simulink model "ASK_SIM"  (R2024a)
settings: Solver=VariableStepAuto  StartTime=0.0  StopTime=10.0  RelTol=1e-3
libraries: commrandsrc3 x1
settings Model: Creator=adity  LastModifiedBy=adity

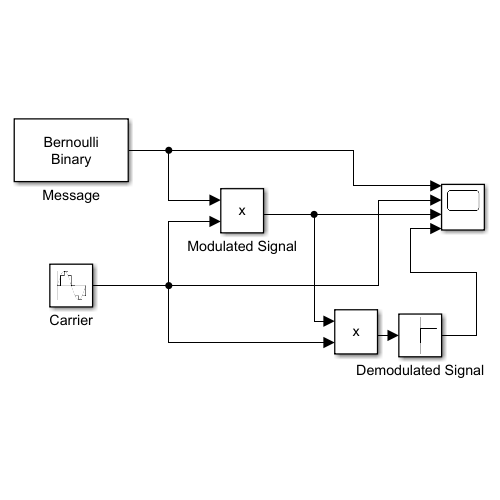
[thumbnail: Simulink's stored preview of the top-level diagram]
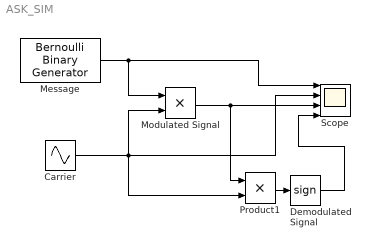
== system ASK_SIM ==
  Carrier : Sin  Frequency=2*pi*5  SampleTime=1/1000  VectorParams1D=off
  Demodulated Signal : Signum
  Message : commrandsrc3/Bernoulli Binary Generator  ProbabilityOfZero=0.5  SeedSource=Auto  Seed=0  SampleTime=0.5  SamplesPerFrame=1  OutputDataType=double  SimulateUsing=Interpreted execution
  Modulated Signal : Product
  Product1 : Product
  Scope : Scope  NumInputPorts=4
  wires:
  Message/1 -> Scope/1, Modulated Signal/1
  Carrier/1 -> Product1/2, Scope/2, Modulated Signal/2
  Modulated Signal/1 -> Product1/1, Scope/3
  Product1/1 -> Demodulated Signal/1
  Demodulated Signal/1 -> Scope/4
